simulink model "thirteen"  (R2022a)
settings: Solver=ode4  StartTime=0.0  StopTime=20  FixedStep=Ts  RelTol=1e-3
InitFcn:
  | Parameter;
values from neighbouring files (symbols this model uses):
  ActuatorDelay = 0.2    [Parameter.m]
  Sampling_time_angle = 0.005    [Parameter.m]
  Sampling_time_distance = 0.01    [Parameter.m]
undefined symbols (not defined in the file or in its folder): DiscIntNeverNeededParam, inertia, initial_condition, motor, trim
libraries: simulink x6, slpidlib x1
settings Model: Creator=wngud  LastModifiedBy=wngud
settings DataIOCC: SaveFinalState=on  SaveFormat=Array  SaveState=on
settings DebuggingCC: UnconnectedInputMsg=warning  UnconnectedOutputMsg=warning  UnconnectedLineMsg=warning
settings RTWCC: DLArmComputeVersion=19.05

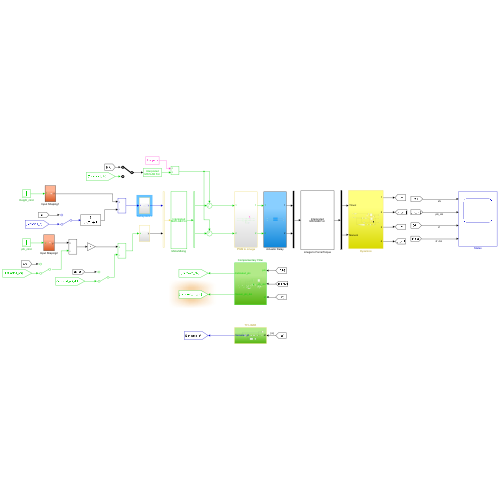
[thumbnail: Simulink's stored preview of the top-level diagram]
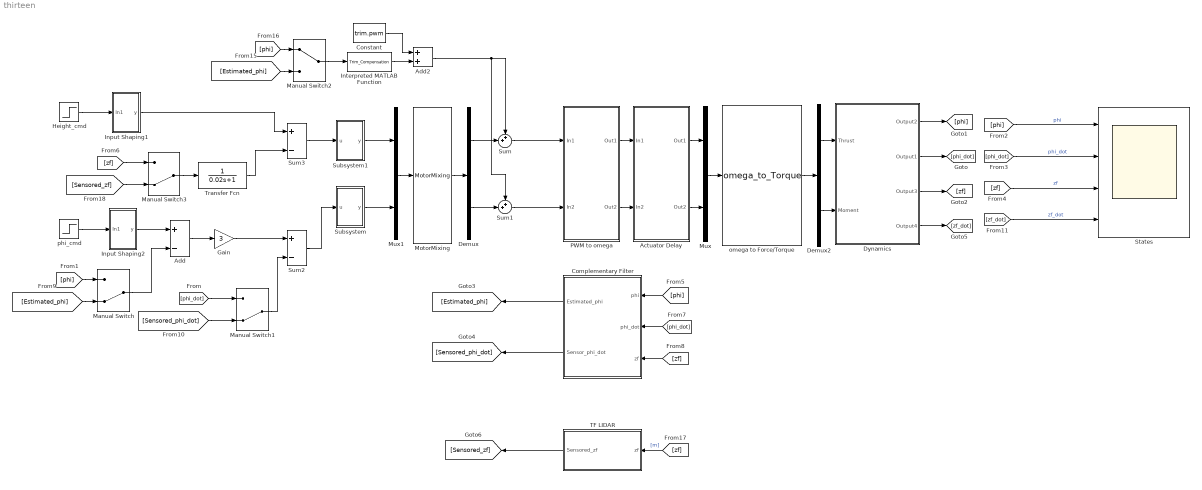
== system thirteen ==
  Actuator Delay : Subsystem
  Add : Sum  Inputs=+-
  Add2 : Sum
  Complementary Filter : Subsystem
  Constant : Constant  Value=trim.pwm
  Demux : Demux  Outputs=2
  Demux2 : Demux  Outputs=2
  Dynamics : Subsystem
  Gain : Gain  Gain=3
  Height_cmd : Step  Time=3  After=0.2  SampleTime=Sampling_time_angle
  Input Shaping1 : Subsystem
  Input Shaping2 : Subsystem
  Interpreted MATLAB Function : MATLABFcn  MATLABFcn=Trim_Compensation  OutputSignalType=real  SampleTime=Sampling_time_angle
  Manual Switch : ManualSwitch  CurrentSetting=0  SampleTime=Sampling_time_angle
  Manual Switch1 : ManualSwitch  CurrentSetting=0  SampleTime=Sampling_time_angle
  Manual Switch2 : ManualSwitch
  Manual Switch3 : ManualSwitch  CurrentSetting=0  SampleTime=Sampling_time_distance
  MotorMixing : MATLABFcn  MATLABFcn=MotorMixing  SampleTime=Sampling_time_angle
  Mux : Mux  Inputs=2
  Mux1 : Mux  Inputs=2
  PWM to omega : Subsystem
  States : Scope  NumInputPorts=4
  Subsystem : Subsystem
  Subsystem1 : Subsystem
  Sum : Sum  Inputs=++|
  Sum1 : Sum  Inputs=++|
  Sum2 : Sum  Inputs=+-  SampleTime=Sampling_time_angle
  Sum3 : Sum  Inputs=+-  SampleTime=Sampling_time_distance
  TF LIDAR : Subsystem
  Transfer Fcn : TransferFcn  Denominator=[0.02 1]
  omega to Force/Torque : MATLABFcn  MATLABFcn=omega_to_Torque
  phi_cmd : Step  Time=0  After=0  SampleTime=Sampling_time_angle  VectorParams1D=off
  wires:
  Actuator Delay/1(Out1) -> Mux/1
  PWM to omega/2(Out2) -> Actuator Delay/2(In2)
  Actuator Delay/2(Out2) -> Mux/2
  PWM to omega/1(Out1) -> Actuator Delay/1(In1)
  Mux/1 -> omega to Force/Torque/1
  omega to Force/Torque/1 -> Demux2/1
  MotorMixing/1 -> Demux/1
  Dynamics/2(Output1) -> [phi_dot]
  Dynamics/3(Output3) -> [zf]
  Dynamics/1(Output2) -> [phi]
  [phi] -> States/1  "phi"
  [phi_dot] -> States/2  "phi_dot"
  [zf] -> States/3  "zf"
  Sum3/1 -> Subsystem1/1(u)
  Sum2/1 -> Subsystem/1(u)
  Gain/1 -> Sum2/1
  Add/1 -> Gain/1
  [phi] -> Complementary Filter/1(phi)
  [phi_dot] -> Complementary Filter/2(phi_dot)
  [zf] -> Complementary Filter/3(zf)
  Complementary Filter/1(Estimated_phi) -> [Estimated_phi]
  Complementary Filter/2(Sensor_phi_dot) -> [Sensored_phi_dot]
  [phi] -> Manual Switch/1
  [Estimated_phi] -> Manual Switch/2
  [phi_dot] -> Manual Switch1/1
  [Sensored_phi_dot] -> Manual Switch1/2
  Manual Switch1/1 -> Sum2/2
  Manual Switch/1 -> Add/2
  [zf_dot] -> States/4  "zf_dot"
  Mux1/1 -> MotorMixing/1
  Demux/1 -> Sum/2
  Demux/2 -> Sum1/2
  [phi] -> Manual Switch2/1
  [Estimated_phi] -> Manual Switch2/2
  Manual Switch2/1 -> Interpreted MATLAB Function/1
  Constant/1 -> Add2/1
  Interpreted MATLAB Function/1 -> Add2/2
  Demux2/1 -> Dynamics/1(Thrust)
  Demux2/2 -> Dynamics/2(Moment)
  Dynamics/4(Output4) -> [zf_dot]
  Sum/1 -> PWM to omega/1(In1)
  Sum1/1 -> PWM to omega/2(In2)
  Subsystem/1(y) -> Mux1/2
  Height_cmd/1 -> Input Shaping1/1(In1)
  Input Shaping1/1(y) -> Sum3/1
  phi_cmd/1 -> Input Shaping2/1(In1)
  Subsystem1/1(y) -> Mux1/1
  [zf] -> TF LIDAR/1(zf)  "[m]"
  TF LIDAR/1(Sensored_zf) -> [Sensored_zf]
  [Sensored_zf] -> Manual Switch3/2
  [zf] -> Manual Switch3/1
  Manual Switch3/1 -> Transfer Fcn/1
  Transfer Fcn/1 -> Sum3/2
  Add2/1 -> Sum1/1, Sum/1
  Input Shaping2/1(y) -> Add/1

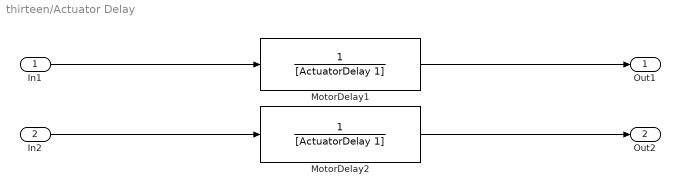
== system thirteen/Actuator Delay ==
  In1 : Inport  SampleTime=Sampling_time_angle
  In2 : Inport  Port=2  SampleTime=Sampling_time_angle
  MotorDelay1 : TransferFcn  Denominator=[ActuatorDelay 1]
  MotorDelay2 : TransferFcn  Denominator=[ActuatorDelay 1]
  Out1 : Outport
  Out2 : Outport  Port=2
  wires:
  In1/1 -> MotorDelay1/1
  MotorDelay2/1 -> Out2/1
  MotorDelay1/1 -> Out1/1
  In2/1 -> MotorDelay2/1

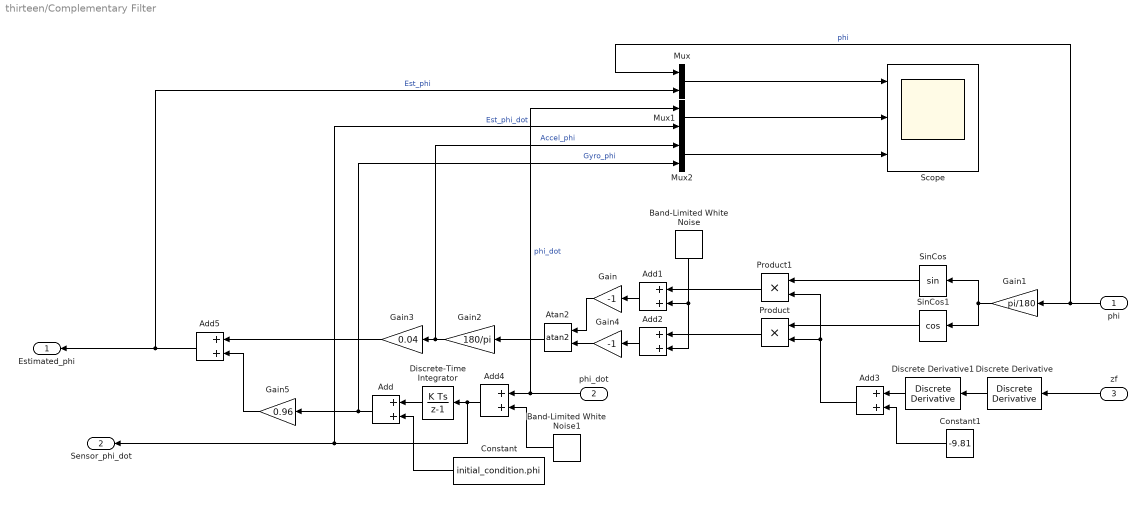
== system thirteen/Complementary Filter ==
  phi : Inport  SampleTime=Sampling_time_angle
  phi_dot : Inport  Port=2  SampleTime=Sampling_time_angle
  zf : Inport  Port=3  SampleTime=Sampling_time_angle
  Add{,1..5} (6 alike) : Sum
  Atan2 : Trigonometry  Operator=atan2
  Band-Limited White Noise : simulink/Sources/Band-Limited White Noise  Cov=0.001  Ts=Sampling_time_angle  seed=[23341]
  Band-Limited White Noise1 : simulink/Sources/Band-Limited White Noise  Cov=0.0001  Ts=Sampling_time_angle  seed=[23341]
  Constant : Constant  Value=initial_condition.phi
  Constant1 : Constant  Value=-9.81
  Discrete Derivative : simulink/Discrete/Discrete Derivative  gainval=1.0  ICPrevScaledInput=0.0  OutMin=[]  OutMax=[]  OutDataType=fixdt(1, 16)  OutScaling=2^-10  DoSatur=off
  Discrete Derivative1 : simulink/Discrete/Discrete Derivative  gainval=1.0  ICPrevScaledInput=0.0  OutMin=[]  OutMax=[]  OutDataType=fixdt(1, 16)  OutScaling=2^-10  DoSatur=off
  Discrete-Time Integrator : DiscreteIntegrator  SampleTime=Sampling_time_angle  ICPrevOutput=DiscIntNeverNeededParam  ICPrevScaledInput=DiscIntNeverNeededParam
  Gain : Gain  Gain=-1
  Gain1 : Gain  Gain=pi/180
  Gain2 : Gain  Gain=180/pi
  Gain3 : Gain  Gain=0.04
  Gain4 : Gain  Gain=-1
  Gain5 : Gain  Gain=0.96
  Mux : Mux  Inputs=2
  Mux1 : Mux  Inputs=2
  Mux2 : Mux  Inputs=2
  Product : Product
  Product1 : Product
  Scope : Scope  NumInputPorts=3
  SinCos : Trigonometry
  SinCos1 : Trigonometry  Operator=cos
  Estimated_phi : Outport
  Sensor_phi_dot : Outport  Port=2
  wires:
  Gain1/1 -> SinCos/1, SinCos1/1
  SinCos/1 -> Product1/1
  Add4/1 -> Discrete-Time Integrator/1, Sensor_phi_dot/1, Mux1/2  "Est_phi_dot"
  Add3/1 -> Product1/2, Product/2
  Gain3/1 -> Add5/1
  Product1/1 -> Add1/1
  Band-Limited White Noise1/1 -> Add4/2
  Gain5/1 -> Add5/2
  Gain2/1 -> Mux2/1, Gain3/1  "Accel_phi"
  Product/1 -> Add2/1
  Band-Limited White Noise/1 -> Add1/2, Add2/2
  phi/1 -> Gain1/1, Mux/1  "phi"
  Atan2/1 -> Gain2/1
  Constant1/1 -> Add3/2
  SinCos1/1 -> Product/1
  Add5/1 -> Estimated_phi/1, Mux/2  "Est_phi"
  phi_dot/1 -> Mux1/1, Add4/1  "phi_dot"
  Add1/1 -> Gain/1
  Gain/1 -> Atan2/1
  Mux/1 -> Scope/1
  Mux1/1 -> Scope/2
  Discrete-Time Integrator/1 -> Add/1
  Add/1 -> Mux2/2, Gain5/1  "Gyro_phi"
  Constant/1 -> Add/2
  Add2/1 -> Gain4/1
  Gain4/1 -> Atan2/2
  Mux2/1 -> Scope/3
  Discrete Derivative1/1 -> Add3/1
  Discrete Derivative/1 -> Discrete Derivative1/1
  zf/1 -> Discrete Derivative/1

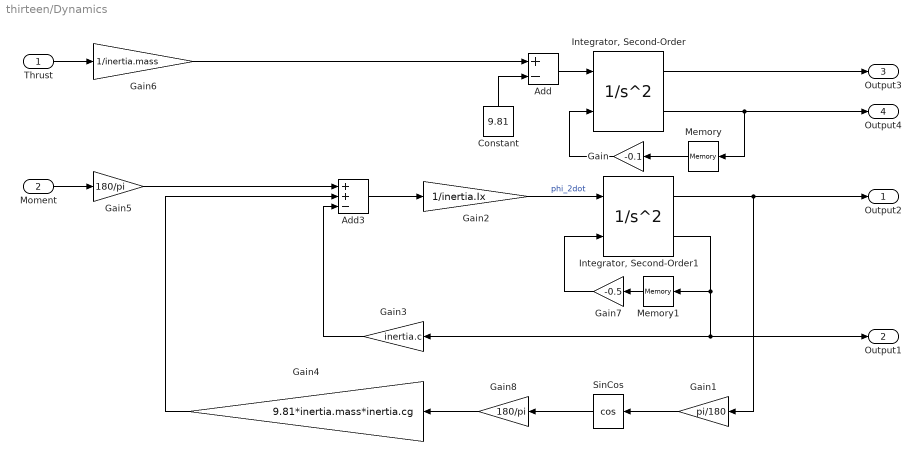
== system thirteen/Dynamics ==
  Thrust : Inport
  Moment : Inport  Port=2
  Add : Sum  Inputs=+-
  Add3 : Sum  Inputs=++-
  Constant : Constant  Value=9.81
  Gain : Gain  Gain=-0.1
  Gain1 : Gain  Gain=pi/180
  Gain2 : Gain  Gain=1/inertia.Ix
  Gain3 : Gain  Gain=inertia.c
  Gain4 : Gain  Gain=9.81*inertia.mass*inertia.cg
  Gain5 : Gain  Gain=180/pi
  Gain6 : Gain  Gain=1/inertia.mass
  Gain7 : Gain  Gain=-0.5
  Gain8 : Gain  Gain=180/pi
  "Integrator, Second-Order" : SecondOrderIntegrator  ICX=initial_condition.zf  LimitX=on  UpperLimitX=10  LowerLimitX=0  StateNameX="\"zf\""  ICSourceDXDT=external  StateNameDXDT="\"zf_dot\""  ReinitDXDTwhenXreachesSaturation=on
  "Integrator, Second-Order1" : SecondOrderIntegrator  ICX=initial_condition.phi  LimitX=on  UpperLimitX=25  LowerLimitX=-25  StateNameX="\"phi\""  ICSourceDXDT=external  StateNameDXDT="\"phi_dot\""  ReinitDXDTwhenXreachesSaturation=on
  Memory : Memory
  Memory1 : Memory
  SinCos : Trigonometry  Operator=cos
  Output2 : Outport
  Output1 : Outport  Port=2
  Output3 : Outport  Port=3
  Output4 : Outport  Port=4
  wires:
  Gain2/1 -> "Integrator, Second-Order1"/1  "phi_2dot"
  "Integrator, Second-Order"/1 -> Output3/1
  Thrust/1 -> Gain6/1
  "Integrator, Second-Order1"/1 -> Output2/1, Gain1/1
  Add3/1 -> Gain2/1
  Gain3/1 -> Add3/3
  "Integrator, Second-Order"/2 -> Output4/1, Memory/1
  Gain/1 -> "Integrator, Second-Order"/2
  Memory/1 -> Gain/1
  "Integrator, Second-Order1"/2 -> Memory1/1, Output1/1, Gain3/1
  Gain6/1 -> Add/1
  Add/1 -> "Integrator, Second-Order"/1
  Constant/1 -> Add/2
  Moment/1 -> Gain5/1
  Memory1/1 -> Gain7/1
  Gain7/1 -> "Integrator, Second-Order1"/2
  Gain1/1 -> SinCos/1
  Gain5/1 -> Add3/1
  SinCos/1 -> Gain8/1
  Gain8/1 -> Gain4/1
  Gain4/1 -> Add3/2

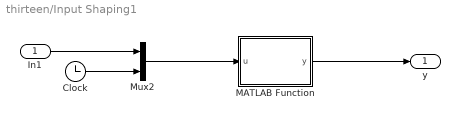
== system thirteen/Input Shaping1 ==
  In1 : Inport
  Clock : Clock
  MATLAB Function : MATLAB Function  TreatAsAtomicUnit=on
  Mux2 : Mux  Inputs=2
  y : Outport
  wires:
  Clock/1 -> Mux2/2
  Mux2/1 -> MATLAB Function/1(u)
  In1/1 -> Mux2/1
  MATLAB Function/1(y) -> y/1

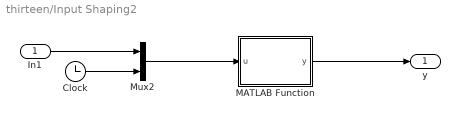
== system thirteen/Input Shaping2 ==
  In1 : Inport
  Clock : Clock
  MATLAB Function : MATLAB Function  TreatAsAtomicUnit=on
  Mux2 : Mux  Inputs=2
  y : Outport
  wires:
  Mux2/1 -> MATLAB Function/1(u)
  Clock/1 -> Mux2/2
  In1/1 -> Mux2/1
  MATLAB Function/1(y) -> y/1

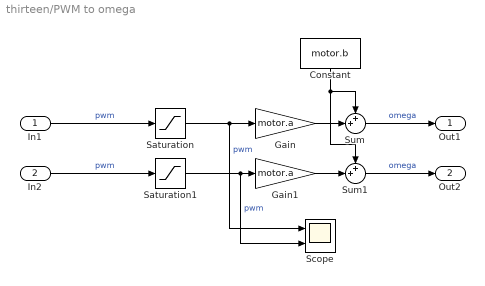
== system thirteen/PWM to omega ==
  In1 : Inport
  In2 : Inport  Port=2
  Constant : Constant  Value=motor.b
  Gain : Gain  Gain=motor.a
  Gain1 : Gain  Gain=motor.a
  Saturation : Saturate  UpperLimit=1900  LowerLimit=1050  RndMeth=Ceiling
  Saturation1 : Saturate  UpperLimit=1900  LowerLimit=1050
  Scope : Scope  NumInputPorts=2
  Sum : Sum  Inputs=++|
  Sum1 : Sum  Inputs=++|
  Out1 : Outport
  Out2 : Outport  Port=2
  wires:
  Gain/1 -> Sum/2
  Constant/1 -> Sum1/1, Sum/1
  Gain1/1 -> Sum1/2
  Sum/1 -> Out1/1  "omega"
  Sum1/1 -> Out2/1  "omega"
  In1/1 -> Saturation/1  "pwm"
  Saturation/1 -> Scope/1, Gain/1  "pwm"
  Saturation1/1 -> Scope/2, Gain1/1  "pwm"
  In2/1 -> Saturation1/1  "pwm"

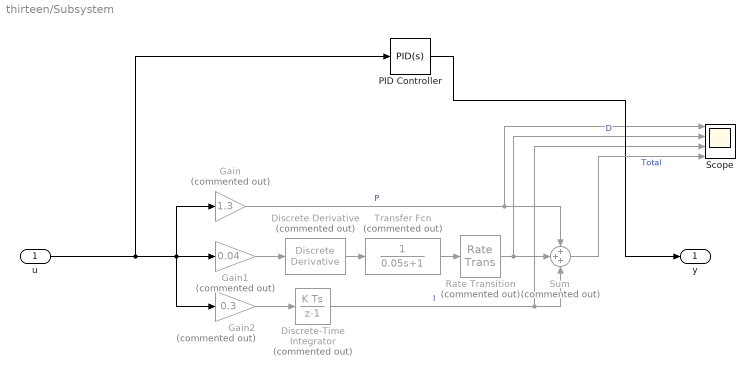
== system thirteen/Subsystem ==
  u : Inport
  Discrete Derivative : simulink/Discrete/Discrete Derivative  Commented=on  gainval=1.0  ICPrevScaledInput=0.0  OutMin=[]  OutMax=[]  OutDataType=fixdt(1, 16)  OutScaling=2^-10  DoSatur=off
  Discrete-Time Integrator : DiscreteIntegrator  Commented=on  SampleTime=Sampling_time_angle  ICPrevOutput=DiscIntNeverNeededParam  ICPrevScaledInput=DiscIntNeverNeededParam
  Gain : Gain  Commented=on  Gain=1.3
  Gain1 : Gain  Commented=on  Gain=0.04
  Gain2 : Gain  Commented=on  Gain=0.3
  PID Controller : slpidlib/PID Controller  Controller=PID  Form=Parallel  TimeDomain=Continuous-time  UseExternalTs=off  SampleTime=Sampling_time_angle  IntegratorMethod=Forward Euler  FilterMethod=Forward Euler  ControllerParametersSource=internal  P=1.3  I=0.3  UseKiTs=off  D=0.04  N=20  UseFilter=on  TunerSelectOption=Transfer Function Based (PID Tuner App)  InitialConditionSource=internal  InitialConditionForIntegrator=0  InitialConditionForFilter=0  DifferentiatorICPrevScaledInput=0  ExternalReset=none  TrackingMode=off  Kt=1  LimitOutput=off  SatLimitsSource=internal  UpperSaturationLimit=inf  LowerSaturationLimit=-inf  LinearizeAsGain=on  AntiWindupMode=none  Kb=1  POutMin=[]  POutMax=[]  IOutMin=[]  IOutMax=[]  DOutMin=[]  DOutMax=[]  NOutMin=[]  NOutMax=[]  SumOutMin=[]  SumOutMax=[]  SaturationOutMin=[]  SaturationOutMax=[]  PParamMin=[]  PParamMax=[]  IParamMin=[]  IParamMax=[]  DParamMin=[]  DParamMax=[]  NParamMin=[]  NParamMax=[]  KbParamMin=[]  KbParamMax=[]  KtParamMin=[]  KtParamMax=[]  KbOutMin=[]  KbOutMax=[]  KtOutMin=[]  KtOutMax=[]  IntegratorOutMin=[]  IntegratorOutMax=[]  FilterOutMin=[]  FilterOutMax=[]  SumI1OutMin=[]  SumI1OutMax=[]  SumI2OutMin=[]  SumI2OutMax=[]  SumI3OutMin=[]  SumI3OutMax=[]  SumI4OutMin=[]  SumI4OutMax=[]  SumDOutMin=[]  SumDOutMax=[]  DifferentiatorOutMin=[]  DifferentiatorOutMax=[]  FilterDiffOutCoefMin=[]  FilterDiffOutCoefMax=[]  ReciprocalOutMin=[]  ReciprocalOutMax=[]  SumDenOutMin=[]  SumDenOutMax=[]  SumNumOutMin=[]  SumNumOutMax=[]  DivideOutMin=[]  DivideOutMax=[]  UdiffTsProdOutMin=[]  UdiffTsProdOutMax=[]  NTsProdOutMin=[]  NTsProdOutMax=[]  UintegralTsProdOutMin=[]  UintegralTsProdOutMax=[]  UngainTsProdOutMin=[]  UngainTsProdOutMax=[]  IntegratorContinuousStateAttributes=''  IntegratorStateMustResolveToSignalObject=off  IntegratorRTWStateStorageClass=Auto  FilterContinuousStateAttributes=''  FilterStateMustResolveToSignalObject=off  FilterRTWStateStorageClass=Auto  ParallelPVariant=InternalParameters  IdealPVariant=Disabled  IVariant=InternalParameters  DVariant=InternalParameters  IntegratorVariant=Continuous  SatVariant=Disabled  AWVariant=Passthrough  PCopyVariant=Disabled  TRVariant=Disabled  FdbkBlocksVariant=Forward  IdealPFdbkVariant=Disabled  SatFdbkVariant=Disabled  DerivativeFilterVariant=ContFilter  NVariant=InternalParameters  NCopyVariant=Disabled  FilterICVariant=InternalICsFilter  IntegratorICVariant=InternalICs  ExternalResetVariant=Disabled  TRSumVariant=Passthrough  SumFdbkVariant=Disabled  SumVariant=Sum_PID  TsampFilterVariant=InternalTs  TsampNgainVariant=Passthrough  TsampIntegralVariant=Passthrough  ExternalSaturationOutDataTypeStr=Inherit: Same as second input  aMode=0
  Rate Transition : RateTransition  Commented=on  OutPortSampleTime=Sampling_time_angle
  Scope : Scope  NumInputPorts=4
  Sum : Sum  Commented=on  Inputs=+++
  Transfer Fcn : TransferFcn  Commented=on  Denominator=[0.05 1]
  y : Outport
  wires:
  Gain1/1 -> Discrete Derivative/1
  Gain2/1 -> Discrete-Time Integrator/1
  Discrete-Time Integrator/1 -> Scope/3, Sum/3  "I"
  Gain/1 -> Scope/1, Sum/1  "P"
  Discrete Derivative/1 -> Transfer Fcn/1
  Transfer Fcn/1 -> Rate Transition/1
  u/1 -> PID Controller/1, Gain/1, Gain2/1, Gain1/1
  Rate Transition/1 -> Scope/2, Sum/2  "D"
  PID Controller/1 -> y/1
  Sum/1 -> Scope/4  "Total"

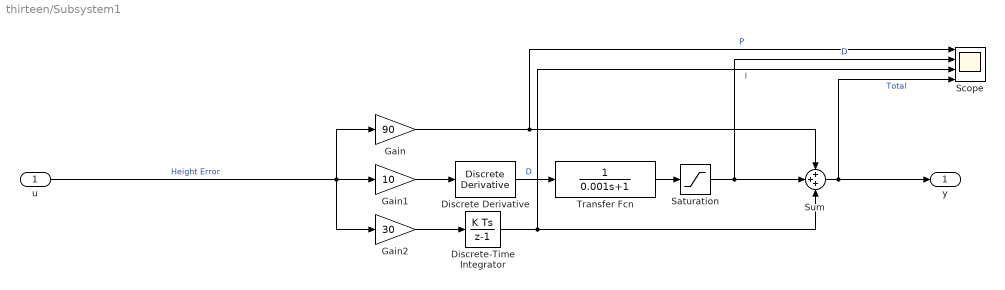
== system thirteen/Subsystem1 ==
  u : Inport  SampleTime=Sampling_time_distance
  Discrete Derivative : simulink/Discrete/Discrete Derivative  gainval=1.0  ICPrevScaledInput=0.0  OutMin=[]  OutMax=[]  OutDataType=fixdt(1, 16)  OutScaling=2^-10  DoSatur=off
  Discrete-Time Integrator : DiscreteIntegrator  SampleTime=Sampling_time_distance  ICPrevOutput=DiscIntNeverNeededParam  ICPrevScaledInput=DiscIntNeverNeededParam
  Gain : Gain  Gain=90
  Gain1 : Gain  Gain=10
  Gain2 : Gain  Gain=30
  Saturation : Saturate  UpperLimit=10  LowerLimit=-10  SampleTime=Sampling_time_distance
  Scope : Scope  NumInputPorts=4
  Sum : Sum  Inputs=+++  SampleTime=Sampling_time_distance
  Transfer Fcn : TransferFcn  Denominator=[0.001 1]
  y : Outport  SampleTime=Sampling_time_distance
  wires:
  Gain2/1 -> Discrete-Time Integrator/1
  Discrete-Time Integrator/1 -> Scope/3, Sum/3  "I"
  Gain/1 -> Scope/1, Sum/1  "P"
  Discrete Derivative/1 -> Transfer Fcn/1  "D"
  u/1 -> Gain/1, Gain2/1, Gain1/1  "Height Error"
  Gain1/1 -> Discrete Derivative/1
  Transfer Fcn/1 -> Saturation/1
  Saturation/1 -> Scope/2, Sum/2  "D"
  Sum/1 -> y/1, Scope/4  "Total"

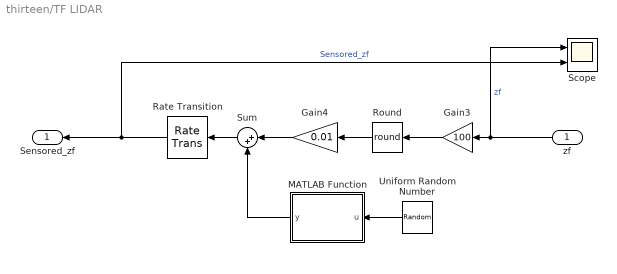
== system thirteen/TF LIDAR ==
  zf : Inport
  Gain3 : Gain  Gain=100
  Gain4 : Gain  Gain=0.01
  MATLAB Function : MATLAB Function  TreatAsAtomicUnit=on
  Rate Transition : RateTransition  OutPortSampleTime=Sampling_time_distance
  Round : Rounding  Operator=round
  Scope : Scope  NumInputPorts=2
  Sum : Sum  Inputs=|++
  Uniform Random Number : UniformRandomNumber  Minimum=0  Seed=2331  SampleTime=Sampling_time_distance
  Sensored_zf : Outport
  wires:
  Round/1 -> Gain4/1
  Gain3/1 -> Round/1
  zf/1 -> Scope/1, Gain3/1  "zf"
  Rate Transition/1 -> Sensored_zf/1, Scope/2  "Sensored_zf"
  Gain4/1 -> Sum/1
  Sum/1 -> Rate Transition/1
  Uniform Random Number/1 -> MATLAB Function/1(u)
  MATLAB Function/1(y) -> Sum/2

== matlab function thirteen/TF LIDAR/MATLAB Function ==
  data: u input; y output
function y = fcn(u)

if u >= 0.99
    y = 0.01;
elseif u <= 0.01
    y = -0.01;
else
    y = 0;
end

== matlab function thirteen/Input Shaping2/MATLAB Function ==
  data: u input; y output
function y = fcn(u)

value       = u(1); % [step size]
time        = u(2); % [sec]
rising_time = 0.5;  % [sec]

y = value*(1-cos(pi/rising_time*(time)))/2;
    
if (time >= rising_time)
    y = value;
end

== matlab function thirteen/Input Shaping1/MATLAB Function ==
  data: u input; y output
function y = fcn(u)

value       = u(1); % [step size]
time        = u(2); % [sec]
rising_time = 0.5;  % [sec]

y = value*(1-cos(pi/rising_time*(time-3)))/2;
    
if (time >= 3 + rising_time)
    y = value;
end
